simulink model "Week1problem3"  (R2020b)
settings: Solver=VariableStepAuto  StartTime=0.0  StopTime=10.0  RelTol=1e-3
settings Model: Creator=Admin  LastModifiedBy=Admin

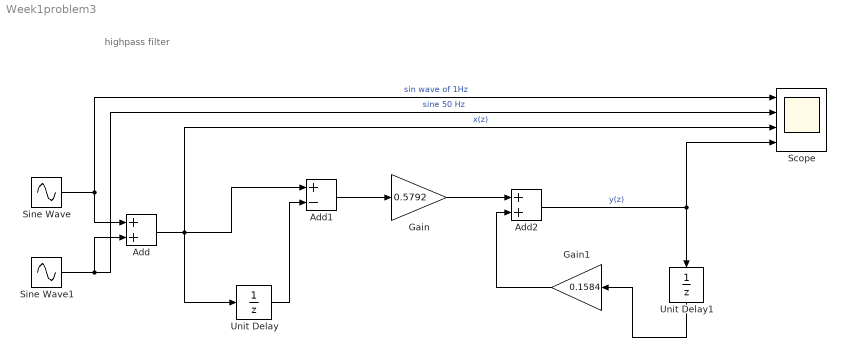
== system Week1problem3 ==
  note: highpass filter
  Add : Sum
  Add1 : Sum  Inputs=+-
  Add2 : Sum
  Gain : Gain  Gain=0.5792
  Gain1 : Gain  Gain=0.1584
  Scope : Scope  NumInputPorts=4
  Sine Wave : Sin  SampleTime=0
  Sine Wave1 : Sin  Frequency=50  SampleTime=0
  Unit Delay : UnitDelay  SampleTime=-1  HasFrameUpgradeWarning=on
  Unit Delay1 : UnitDelay  SampleTime=-1  HasFrameUpgradeWarning=on
  wires:
  Sine Wave/1 -> Add/1, Scope/1  "sin wave of 1Hz"
  Sine Wave1/1 -> Scope/2, Add/2  "sine 50 Hz"
  Add/1 -> Scope/3, Unit Delay/1, Add1/1  "x(z)"
  Unit Delay/1 -> Add1/2
  Add1/1 -> Gain/1
  Gain/1 -> Add2/1
  Gain1/1 -> Add2/2
  Unit Delay1/1 -> Gain1/1
  Add2/1 -> Scope/4, Unit Delay1/1  "y(z)"
